simulink model "ControlPC_XBOX"  (R2025a)
settings: Solver=FixedStepDiscrete  StartTime=0.0  StopTime=inf  FixedStep=0.01  RelTol=1e-3
libraries: simulink x1, instrumentlib x1
settings Model: SILPILModeSetting=veronly  Creator=pablo  LastModifiedBy=aj
settings SolverCC: AutoInsertRateTranBlk=on
settings OptimizationCC: EnhancedBackFolding=on  PassReuseOutputArgsAs=Individual arguments  ZeroExternalMemoryAtStartup=off  ZeroInternalMemoryAtStartup=off  MaxStackSize=64  OptimizeBlockOrder=speed  DifferentSizesBufferReuse=on  OptimizationCustomize=off  EfficientTunableParamExpr=on
settings DebuggingCC: ReadBeforeWriteMsg=DisableAll  WriteAfterWriteMsg=DisableAll  WriteAfterReadMsg=DisableAll  MultiTaskDSMMsg=none  ParameterTunabilityLossMsg=error
settings HardwareCC: ProdBitPerPointer=32.0  ProdBitPerSizeT=32.0  ProdBitPerPtrDiffT=32.0  ProdLargestAtomicInteger=Long  ProdLargestAtomicFloat=Double  ProdWordSize=32.0  ProdHWDeviceType=ARM Compatible->ARM Cortex
settings ModelReferenceCC: UpdateModelReferenceTargets=IfOutOfDate
settings SFSimCC: SFSimEcho=off  MATLABDynamicMemAlloc=off
settings RTWCC: SystemTargetFile=ert.tlc  TemplateMakefile=ert_default_tmf  Toolchain=Arduino ARM  BuildConfiguration=Faster Runs  GPUComputeCapability=3.5  Description=Embedded Coder
settings CodeAppCC: ForceParamTrailComments=on  IgnoreCustomStorageClasses=off  OperatorAnnotations=on  SimulinkDataObjDesc=on  SFDataObjDesc=on  InsertBlockDesc=on
settings ERTTargetCC: ExtModeTransport=3.0  ExtModeStaticAllocSize=8192.0  InlinedParameterPlacement=Hierarchical  ERTCustomFileTemplate=example_file_process.tlc  DynamicArrayContainerType=coder::array  SupportContinuousTime=on  SupportNonInlinedSFcns=on

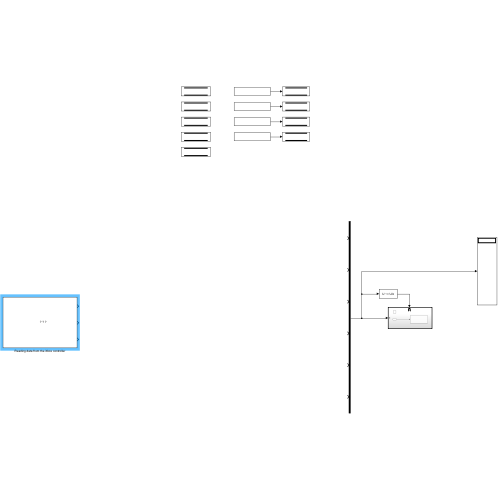
[thumbnail: Simulink's stored preview of the top-level diagram]
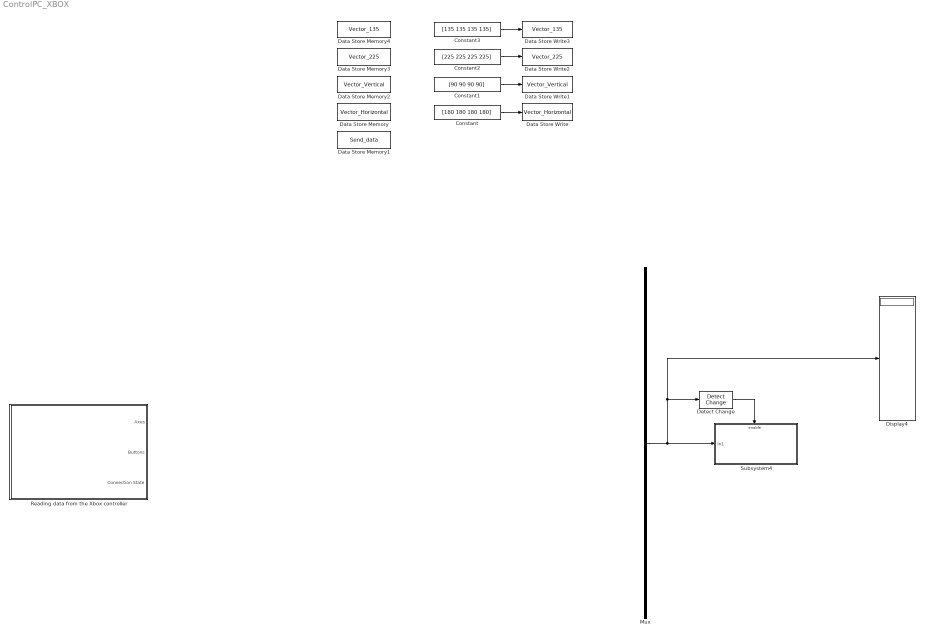
== system ControlPC_XBOX ==
  Constant : Constant  Value=[180 180 180 180]  OutDataTypeStr=int16
  Constant1 : Constant  Value=[90 90 90 90]  OutDataTypeStr=int16
  Constant2 : Constant  Value=[225 225 225 225]  OutDataTypeStr=int16
  Constant3 : Constant  Value=[135 135 135 135]  OutDataTypeStr=int16
  Data Store Memory : DataStoreMemory  DataStoreName=Vector_Horizontal  WriteAfterWriteMsg=warning  ShowAdditionalParam=off  OutDataTypeStr=int16  Dimensions=4
  Data Store Memory1 : DataStoreMemory  DataStoreName=Send_data  WriteAfterWriteMsg=warning  ShowAdditionalParam=off  OutDataTypeStr=int16  Dimensions=4
  Data Store Memory2 : DataStoreMemory  DataStoreName=Vector_Vertical  WriteAfterWriteMsg=warning  ShowAdditionalParam=off  OutDataTypeStr=int16  Dimensions=4
  Data Store Memory3 : DataStoreMemory  DataStoreName=Vector_225  WriteAfterWriteMsg=warning  ShowAdditionalParam=off  OutDataTypeStr=int16  Dimensions=4
  Data Store Memory4 : DataStoreMemory  DataStoreName=Vector_135  WriteAfterWriteMsg=warning  ShowAdditionalParam=off  OutDataTypeStr=int16  Dimensions=4
  Data Store Write : DataStoreWrite  DataStoreName=Vector_Horizontal  IndexOptions=Index vector (dialog)  Indices=1  OutputSizes=1
  Data Store Write1 : DataStoreWrite  DataStoreName=Vector_Vertical  IndexOptions=Index vector (dialog)  Indices=1  OutputSizes=1
  Data Store Write2 : DataStoreWrite  DataStoreName=Vector_225  IndexOptions=Index vector (dialog)  Indices=1  OutputSizes=1
  Data Store Write3 : DataStoreWrite  DataStoreName=Vector_135  IndexOptions=Index vector (dialog)  Indices=1  OutputSizes=1
  Detect Change : simulink/Logic and Bit Operations/Detect Change  vinit=0  OutDataTypeStr=boolean
  Display4 : Display
  Mux : Mux  Inputs=6
  Reading data from the Xbox controller : Subsystem
      mask Display: image('mando.PNG'); % Use "Edit Image" on toolstrip to change.
  Subsystem4 : Subsystem
  wires:
  Constant/1 -> Data Store Write/1
  Constant1/1 -> Data Store Write1/1
  Constant2/1 -> Data Store Write2/1
  Constant3/1 -> Data Store Write3/1
  Mux/1 -> Subsystem4/1(In1), Detect Change/1, Display4/1
  Detect Change/1 -> Subsystem4/Enable

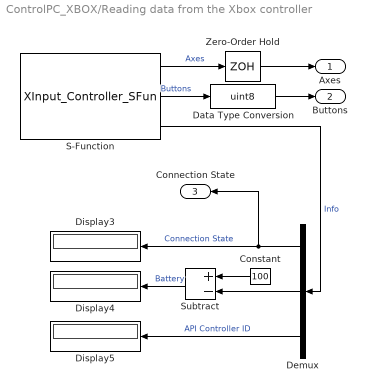
== system ControlPC_XBOX/Reading data from the Xbox controller ==
  Constant : Constant  Value=100
  Data Type Conversion : DataTypeConversion  OutDataTypeStr=uint8  ConvertRealWorld=Stored Integer (SI)  SaturateOnIntegerOverflow=off  RndMeth=Floor
  Demux : Demux  Outputs=3
  Display3 : Display
  Display4 : Display
  Display5 : Display
  S-Function : S-Function  FunctionName=XInput_Controller_SFun  Parameters=ControllerID  SFunctionDeploymentMode=off  EnableBusSupport=off  mask(XInput Controller){ControllerID=1}
      mask help:
      | This Block will allow you to use XInput Controllers in Simulink.
      | XInput is the most Supported API.
      | Works with XBOX 360 and XBOX ONE Controllers.
      |
      | Use 'DEMUX' to access Signals
      | Output_1 [1x6]
      |   Analog Left X, Analog Left Y,
      |   Analog Right X, Analog Right Y,
      |   Left Trigger, Right Trigger
      | Output_2 [1x14]
      |   Up, Down, Left, Right,
      |   Start, Back, Left Stick, Right Stick,
      |   Left Shoulder, Right Shoulder,
      |   A, B, X, Y
      | Output_3 [1x3]
      |   Connection State, Battery Level (1-4), Controller ID
      mask init:
      | ControllerID;   
      | blk = gcb; 
      | get_String = get_param(blk,'ControllerID');
      | ControllerID = str2double(get_String);
      mask Help:
      | Based on Microsoft XInput API
      | Therefore the maximum of conneced Gamepads per PC is 4. First Gamepad has Controller ID 1.
      | 
      | Reference:
      | https://docs.microsoft.com/en-us/windows/win32/api/_xinput/
      | 
      | Tutorial:
      | https://docs.microsoft.com/en-us/windows/win32/xinput/getting-started-with-xinput
      | 
      | Info:
      | The Analog Sticks Deadzone is coded to:
      | Deadzone = 6144;
      | 0 <= Deadzone <= 65534
      | This is smaller then Microsoft default.
      | 
      | created by Mathias Voigt
      | Technische Universität Dresden
      | 2019
      mask TypeOptions ControllerID: 1 | 2 | 3 | 4
      mask DialogControl ParameterGroupVar Prompt: Controller ID
      mask Display:
      | %% Set Block picture from user Data
      | %  (permanent, picture file not needed)
      | %  see persistent_image_allocation.m
      | 
      | %get the picture data
      | UserDataStrut = get_param(gcb, 'UserData');
      | image(UserDataStrut.Image, [0.2, 0.3, 0.6, 0.6])
      | 
      | 
      | 
      | % conventional method (does not save picture data in Simulink)
      | % image('XBOX_One_Controller_Icon.png', [0.2, 0.3, 0.6, 0.6])
      | 
      | %% Create Port Labels
      | color('blue');
      | port_label('output', 1, 'Axes');
      | port_label('output', 2, 'Buttons');
      | port_label('output', 3, 'Info');
      | 
      | 
      | %% Create S-Function Block Name
      | color('black');
      | text(0.5, 0.1, 'XInput Controller',...
      |      'horizontalAlignment', 'center',...
      |      'verticalAlignment', 'bottom');
  Subtract : Sum  Inputs=+-
  Zero-Order Hold : ZeroOrderHold  SampleTime=-1
  Axes : Outport
  Buttons : Outport  Port=2
  Connection State : Outport  Port=3
  wires:
  Demux/1 -> Connection State/1, Display3/1  "Connection State"
  Zero-Order Hold/1 -> Axes/1
  Demux/3 -> Display5/1  "API Controller ID"
  S-Function/1 -> Zero-Order Hold/1  "Axes"
  S-Function/3 -> Demux/1  "Info"
  S-Function/2 -> Data Type Conversion/1  "Buttons"
  Constant/1 -> Subtract/1
  Subtract/1 -> Display4/1  "Battery"
  Demux/2 -> Subtract/2
  Data Type Conversion/1 -> Buttons/1

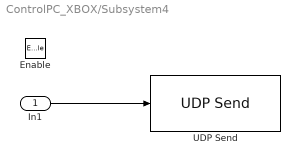
== system ControlPC_XBOX/Subsystem4 ==
  In1 : Inport
  Enable : EnablePort
  UDP Send : instrumentlib/UDP Send  Host=192.168.10.101  Port=8885  LocalAddress=0.0.0.0  LocalPort=-1  EnablePortSharing=off  OutputDatagramPacketSize=18  ByteOrder=little-endian  EnableBlockingMode=on  SimulateUsing=Interpreted execution
  wires:
  In1/1 -> UDP Send/1
